simulink model "Aprendendo_Simulink"  (R2018a)
settings: Solver=VariableStepAuto  StartTime=0.0  StopTime=10  RelTol=1e-3
undefined symbols (not defined in the file or in its folder): a1, f1, fa, Ta
libraries: simulink x2, dspsrcs4 x2, dspsnks4 x1, dsparch4 x1, commseqgen3 x1
settings Model: Creator=marco  LastModifiedBy=marco

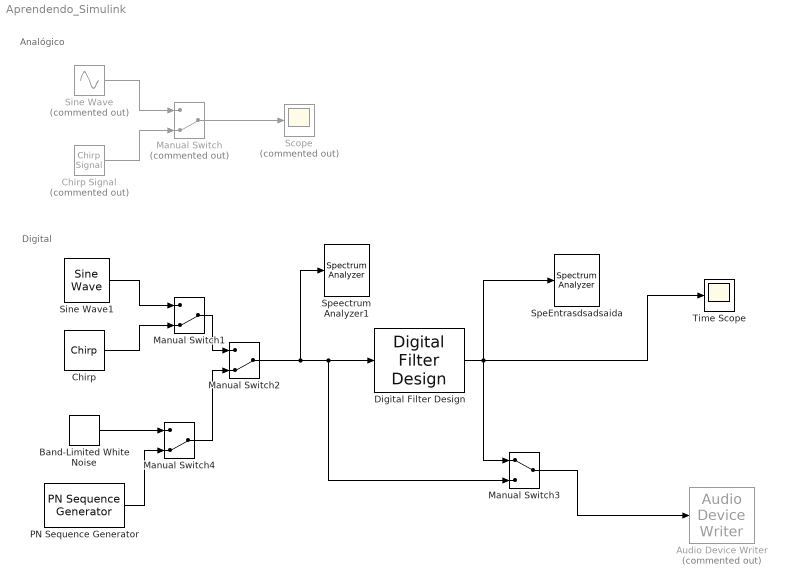
== system Aprendendo_Simulink ==
  note: Digital
  note: Analógico
  Audio Device Writer : dspsnks4/Audio Device Writer  Commented=on  Driver=DirectSound  Device=Default  InheritSampleRate=on  SampleRate=44100  BitDepth=16-bit integer  BufferSize=4096  NumBuffers=10  DefaultOutputChannelMapping=on  OutputChannelMapping=1:2  OutputNumUnderrunSamples=off  DriverIdx=1  DeviceWarnFlag=''
  Band-Limited White Noise : simulink/Sources/Band-Limited White Noise  Cov=[0.1]  Ts=Ta  seed=[23341]
  Chirp : dspsrcs4/Chirp  sweep=Linear  mode=Unidirectional  f0=0  f1=fa/2  t1=1  Tsweep=10  phase=0  Ts=Ta  spf=spf  datatype=Single  OutputFrames=off
      settings: SourceProductName=DSP System Toolbox
  Chirp Signal : simulink/Sources/Chirp Signal  Commented=on  f1=10  T=1  f2=5000
  Digital Filter Design : dsparch4/Digital Filter Design  mwdsp_browser_bugfix_var=off
  Manual Switch : ManualSwitch  Commented=on  CurrentSetting=0
  Manual Switch1 : ManualSwitch  CurrentSetting=0
  Manual Switch2 : ManualSwitch  CurrentSetting=0
  Manual Switch3 : ManualSwitch
  Manual Switch4 : ManualSwitch  CurrentSetting=0
  PN Sequence Generator : commseqgen3/PN Sequence Generator  poly='z^6 + z + 1'  ini_sta=[0 0 0 0 0 1]  outBitMaskSource=Dialog parameter  shift=0  outVarSiz=off  maxOutSizeMode=Dialog parameter  maxOutSize=[10 1]  Ts=1  sampPerFrame=1  reset=off  bitPackedOutputs=off  outDataType=double  numPackedBits=8  bitPackDataSigned=off  bitPackedOutDType=double
      settings: SourceProductName=Communications System Toolbox
  Scope : Scope  Commented=on
  Sine Wave : Sin  Commented=on  Amplitude=10  Bias=5  Frequency=5000*2*pi  Phase=pi/2  SampleTime=0
  Sine Wave1 : dspsrcs4/Sine Wave  Amplitude=a1  Frequency=f1  Phase=0  SampleMode=Discrete  OutComplex=Real  CompMethod=Trigonometric fcn  TableSize=Speed  SampleTime=Ta  SamplesPerFrame=spf  ResetState=Restart at time zero  OutputFrames=off  dataType=double  wordLen=16  udDataType=sfix(16)  fracBitsMode=Best precision  numFracBits=15  OutDataTypeStr=double  LastOutDataTypeStr=double
  "SpeEntrasdsadsaida " : SpectrumAnalyzer
  Speectrum Analyzer1 : SpectrumAnalyzer
  Time Scope : Scope
  wires:
  Sine Wave/1 -> Manual Switch/1
  Chirp Signal/1 -> Manual Switch/2
  Manual Switch/1 -> Scope/1
  Sine Wave1/1 -> Manual Switch1/1
  Chirp/1 -> Manual Switch1/2
  Manual Switch1/1 -> Manual Switch2/1
  Manual Switch2/1 -> Speectrum Analyzer1/1, Manual Switch3/2, Digital Filter Design/1
  Manual Switch3/1 -> Audio Device Writer/1
  Digital Filter Design/1 -> "SpeEntrasdsadsaida "/1, Manual Switch3/1, Time Scope/1
  PN Sequence Generator/1 -> Manual Switch4/2
  Band-Limited White Noise/1 -> Manual Switch4/1
  Manual Switch4/1 -> Manual Switch2/2
